simulink model "PassStBkReclnHolderChk"  (R2018b)
settings: Solver=FixedStepDiscrete  StartTime=0.0  StopTime=10.0  FixedStep=0.01  RelTol=1e-3
libraries: simulink x1
settings Model: Creator=sn2xws  LastModifiedBy=sn2xws
settings Model: ModifiedHistory=|
  | 2024.6.26 V3.0.0 557模式流程
  | 2024.11.6 V3.0.1 V2.6 Md30增加靠背位置1
  | 25.7.4 V3.13.0 新增Md61 Md62
settings DataIOCC: SaveFormat=StructureWithTime
settings OptimizationCC: DefaultParameterBehavior=Inlined  EnhancedBackFolding=on  PassReuseOutputArgsAs=Individual arguments  ZeroExternalMemoryAtStartup=off  ZeroInternalMemoryAtStartup=off  OptimizeBlockOrder=speed  DifferentSizesBufferReuse=on  OptimizationCustomize=off
settings DebuggingCC: ParameterTunabilityLossMsg=error
settings SFSimCC: MATLABDynamicMemAlloc=off
settings RTWCC: SystemTargetFile=autosar.tlc  GenCodeOnly=on  TemplateMakefile=ert_default_tmf  Description=AUTOSAR  GenerateReport=on  IncludeHyperlinkInReport=on  LaunchReport=on  GenerateTraceInfo=on  GenerateTraceReport=on  GenerateTraceReportSl=on  GenerateTraceReportSf=on  GenerateTraceReportEml=on
settings CodeAppCC: ForceParamTrailComments=on  IgnoreCustomStorageClasses=off  OperatorAnnotations=on  SimulinkDataObjDesc=on  SFDataObjDesc=on  InsertBlockDesc=on
settings STFCustomTargetCC: TargetLangStandard=C99 (ISO)  MultiwordLength=256  ParMdlRefBuildCompliant=on  CompOptLevelCompliant=on  IncludeMdlTerminateFcn=off  CombineOutputUpdateFcns=on  SuppressErrorStatus=on  ERTCustomFileBanners=on  SupportNonFinite=off  SupportComplex=off  SupportContinuousTime=off  SupportNonInlinedSFcns=off  RemoveResetFunc=on  MATLABClassNameForMDSCustomization=Simulink.SoftwareTarget.ERTCustomization  AutosarCompliant=on  UseToolchainInfoCompliant=on  LookupTableObjectStructAxisOrder=2,1,3,4,...  LUTObjectStructOrderEvenSpacing=Size,Table,Breakpoints  SystemTargetFile=autosar.tlc
settings ERTTargetCC: TargetLangStandard=C99 (ISO)  ConcurrentExecutionCompliant=off  IncludeMdlTerminateFcn=off  SuppressErrorStatus=on  SupportNonFinite=off  SupportComplex=off  ModelStepFunctionPrototypeControlCompliant=off  CPPClassGenCompliant=off  AutosarCompliant=on  LookupTableObjectStructAxisOrder=2,1,3,4,...  LUTObjectStructOrderEvenSpacing=Size,Table,Breakpoints  InlinedParameterPlacement=NonHierarchical  ERTCustomFileTemplate=example_file_process.tlc  ERTFilePackagingFormat=Compact

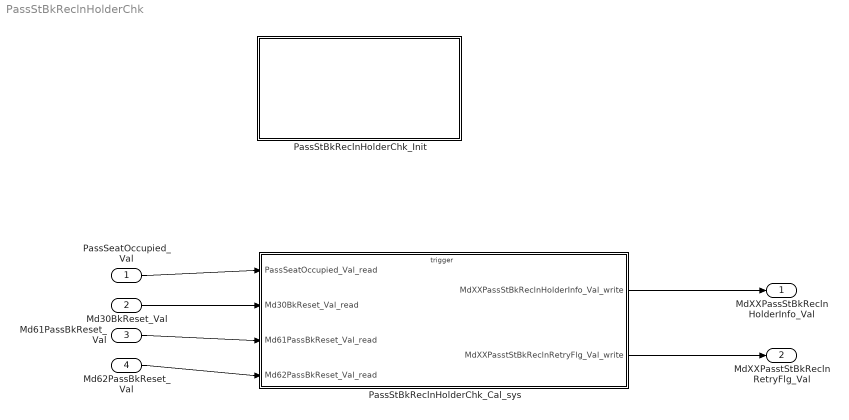
== system PassStBkReclnHolderChk ==
  PassSeatOccupied_Val : Inport  OutDataTypeStr=boolean  PortDimensions=1
  Md30BkReset_Val : Inport  Port=2  OutDataTypeStr=boolean  PortDimensions=1
  Md61PassBkReset_Val : Inport  Port=3  OutDataTypeStr=boolean  PortDimensions=1
  Md62PassBkReset_Val : Inport  Port=4  OutDataTypeStr=boolean  PortDimensions=1
  PassStBkReclnHolderChk_Cal_sys : Subsystem
  PassStBkReclnHolderChk_Init : Subsystem
  MdXXPassStBkReclnHolderInfo_Val : Outport  OutDataTypeStr=uint32  PortDimensions=1
  MdXXPasstStBkReclnRetryFlg_Val : Outport  Port=2  OutDataTypeStr=uint32  PortDimensions=1
  wires:
  PassSeatOccupied_Val/1 -> PassStBkReclnHolderChk_Cal_sys/1(PassSeatOccupied_Val_read)
  PassStBkReclnHolderChk_Cal_sys/1(MdXXPassStBkReclnHolderInfo_Val_write) -> MdXXPassStBkReclnHolderInfo_Val/1
  Md30BkReset_Val/1 -> PassStBkReclnHolderChk_Cal_sys/2(Md30BkReset_Val_read)
  PassStBkReclnHolderChk_Cal_sys/2(MdXXPasstStBkReclnRetryFlg_Val_write) -> MdXXPasstStBkReclnRetryFlg_Val/1
  Md61PassBkReset_Val/1 -> PassStBkReclnHolderChk_Cal_sys/3(Md61PassBkReset_Val_read)
  Md62PassBkReset_Val/1 -> PassStBkReclnHolderChk_Cal_sys/4(Md62PassBkReset_Val_read)

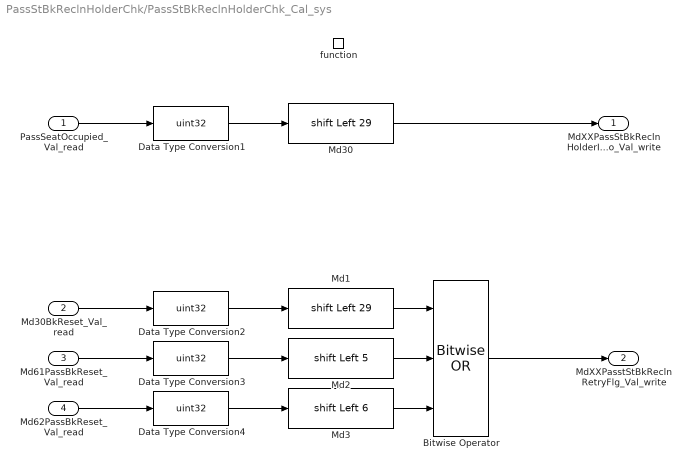
== system PassStBkReclnHolderChk/PassStBkReclnHolderChk_Cal_sys ==
  PassSeatOccupied_Val_read : Inport
  Md30BkReset_Val_read : Inport  Port=2
  Md61PassBkReset_Val_read : Inport  Port=3
  Md62PassBkReset_Val_read : Inport  Port=4
  function : TriggerPort  TriggerType=function-call  IsSimulinkFunction=on  FunctionName=PassStBkReclnHolderChk_Cal  VariantControl=(inherit)
  Bitwise Operator : simulink/Logic and Bit Operations/Bitwise Operator  logicop=OR  UseBitMask=off  NumInputPorts=3  BitMask=bin2dec('11011001')  BitMaskRealWorld=Stored Integer
  Data Type Conversion{1..4} (4 alike) : DataTypeConversion  OutDataTypeStr=uint32
  Md1 : ArithShift  BitShiftNumber=29  BitShiftDirection=Left
  Md2 : ArithShift  BitShiftNumber=5  BitShiftDirection=Left
  Md3 : ArithShift  BitShiftNumber=6  BitShiftDirection=Left
  Md30 : ArithShift  BitShiftNumber=29  BitShiftDirection=Left
  MdXXPassStBkReclnHolderInfo_Val_write : Outport
      settings: EnsureOutportIsVirtual=on
  MdXXPasstStBkReclnRetryFlg_Val_write : Outport  Port=2
      settings: EnsureOutportIsVirtual=on
  wires:
  PassSeatOccupied_Val_read/1 -> Data Type Conversion1/1
  Md30/1 -> MdXXPassStBkReclnHolderInfo_Val_write/1
  Data Type Conversion1/1 -> Md30/1
  Md30BkReset_Val_read/1 -> Data Type Conversion2/1
  Data Type Conversion2/1 -> Md1/1
  Md61PassBkReset_Val_read/1 -> Data Type Conversion3/1
  Md62PassBkReset_Val_read/1 -> Data Type Conversion4/1
  Data Type Conversion3/1 -> Md2/1
  Data Type Conversion4/1 -> Md3/1
  Md1/1 -> Bitwise Operator/1
  Md2/1 -> Bitwise Operator/2
  Md3/1 -> Bitwise Operator/3
  Bitwise Operator/1 -> MdXXPasstStBkReclnRetryFlg_Val_write/1

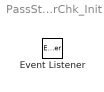
== system PassStBkReclnHolderChk/PassStBkReclnHolderChk_Init ==
  Event Listener : EventListener  EventName=reset
